simulink model "pider"  (R2020b)
settings: Solver=FixedStepAuto  StartTime=0.0  StopTime=30  FixedStep=0.1  RelTol=1e-3
model workspace (MAT data in the model file):
  bbf = [1 -1.905 0.9048]
  licz = [3.944 -7.818 3.874]
values from neighbouring files (symbols this model uses):
  T1 = 0.4    [untitled.m]
  T2 = 0.1    [untitled.m]
undefined symbols (not defined in the file or in its folder): licz1, licz2, mian1, mian2
settings Model: Creator=mbober  LastModifiedBy=mbober

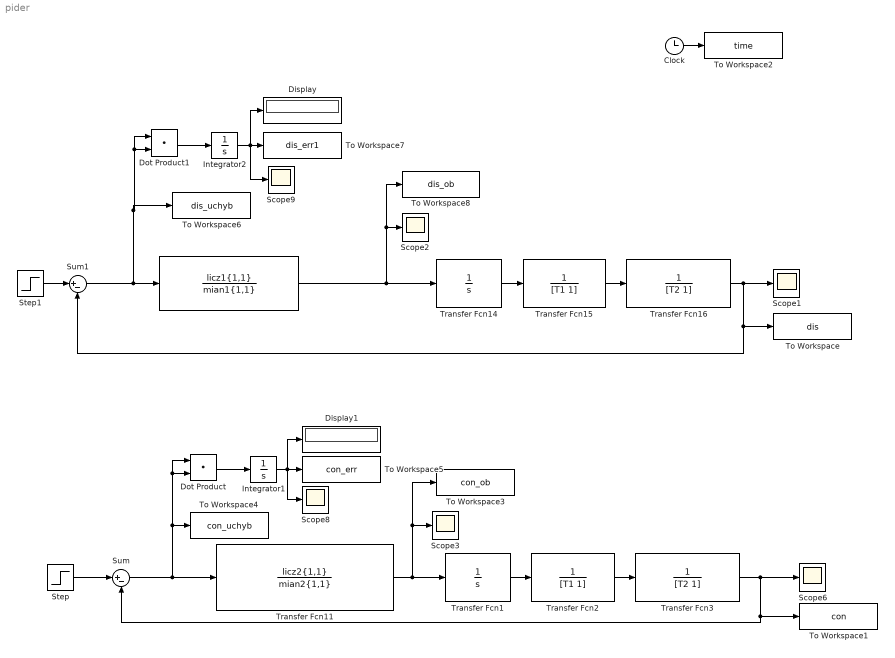
== system pider ==
  " " : DiscreteTransferFcn  Numerator=licz1{1,1}  Denominator=mian1{1,1}
  Clock : Clock
  Display : Display
  Display1 : Display
  Dot Product : DotProduct  InputSameDT=on  OutDataTypeStr=Inherit: Inherit via internal rule
  Dot Product1 : DotProduct  InputSameDT=on  OutDataTypeStr=Inherit: Inherit via internal rule
  Integrator1 : Integrator
  Integrator2 : Integrator
  Scope{1..3,6,8..9} (6 alike) : Scope
  Step : Step  SampleTime=0
  Step1 : Step  SampleTime=0
  Sum : Sum  Inputs=|+-
  Sum1 : Sum  Inputs=|+-
  To Workspace : ToWorkspace  VariableName=dis  SampleTime=-1
  To Workspace1 : ToWorkspace  VariableName=con  SampleTime=-1
  To Workspace2 : ToWorkspace  VariableName=time  SampleTime=-1
  To Workspace3 : ToWorkspace  VariableName=con_ob  SampleTime=-1
  To Workspace4 : ToWorkspace  VariableName=con_uchyb  SampleTime=-1
  To Workspace5 : ToWorkspace  VariableName=con_err  SampleTime=-1
  To Workspace6 : ToWorkspace  VariableName=dis_uchyb  SampleTime=-1
  To Workspace7 : ToWorkspace  VariableName=dis_err1  SampleTime=-1
  To Workspace8 : ToWorkspace  VariableName=dis_ob  SampleTime=-1
  Transfer Fcn1 : TransferFcn  Denominator=[1 0]
  Transfer Fcn11 : TransferFcn  Numerator=licz2{1,1}  Denominator=mian2{1,1}
  Transfer Fcn14 : TransferFcn  Denominator=[1 0]
  Transfer Fcn15 : TransferFcn  Denominator=[T1 1]
  Transfer Fcn16 : TransferFcn  Denominator=[T2 1]
  Transfer Fcn2 : TransferFcn  Denominator=[T1 1]
  Transfer Fcn3 : TransferFcn  Denominator=[T2 1]
  wires:
  Step/1 -> Sum/1
  Transfer Fcn1/1 -> Transfer Fcn2/1
  Transfer Fcn2/1 -> Transfer Fcn3/1
  Transfer Fcn3/1 -> Scope6/1, Sum/2, To Workspace1/1
  Sum/1 -> Transfer Fcn11/1, Dot Product/1, Dot Product/2, To Workspace4/1
  Clock/1 -> To Workspace2/1
  Dot Product/1 -> Integrator1/1
  Integrator1/1 -> To Workspace5/1, Display1/1, Scope8/1
  Integrator2/1 -> Display/1, To Workspace7/1, Scope9/1
  Dot Product1/1 -> Integrator2/1
  Sum1/1 -> " "/1, Dot Product1/1, Dot Product1/2, To Workspace6/1
  Transfer Fcn11/1 -> To Workspace3/1, Scope3/1, Transfer Fcn1/1
  Transfer Fcn16/1 -> Scope1/1, To Workspace/1, Sum1/2
  Transfer Fcn14/1 -> Transfer Fcn15/1
  " "/1 -> Transfer Fcn14/1, To Workspace8/1, Scope2/1
  Transfer Fcn15/1 -> Transfer Fcn16/1
  Step1/1 -> Sum1/1
